simulink model "model"  (R2020b)
settings: Solver=VariableStepAuto  StartTime=0.0  StopTime=20  MaxStep=0.001  RelTol=1e-3
model workspace (MAT data in the model file):
  M1 = Simulink.Parameter
  M1.Value = 100
  M1.DataType = 'auto'
  M1.Dimensions = [1 1]
  b = Simulink.Parameter
  b.Value = 50
  b.DataType = 'auto'
  b.Dimensions = [1 1]
  k1 = Simulink.Parameter
  k1.Value = 50
  k1.DataType = 'auto'
  k1.Dimensions = [1 1]
settings Model: OrderedModelArguments=off  Creator=Lenovo  LastModifiedBy=Lenovo

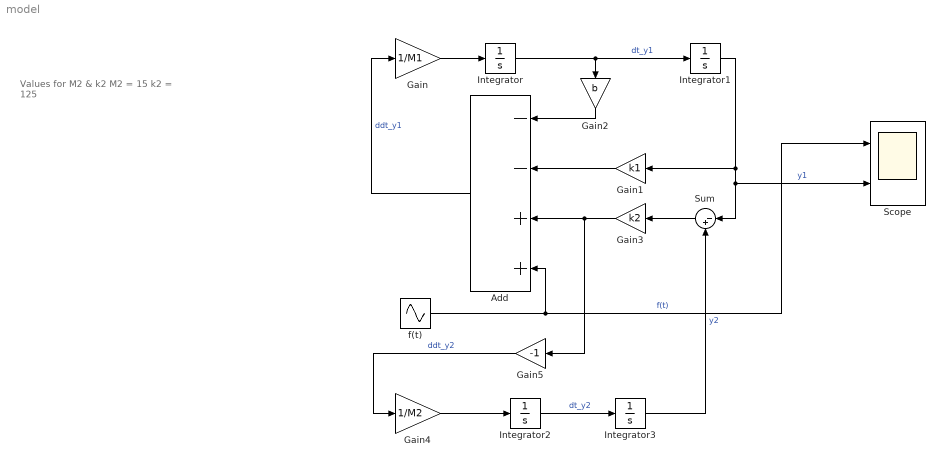
== system model ==
  note: Values for M2 & k2
      | M2 = 15
      | k2 = 125
  Add : Sum  Inputs=--++
  Gain : Gain  Gain=1/M1
  Gain1 : Gain  Gain=k1
  Gain2 : Gain  Gain=b
  Gain3 : Gain  Gain=k2  mask{k2=125}
  Gain4 : Gain  Gain=1/M2  mask{M2=15}
  Gain5 : Gain  Gain=-1
  Integrator{,1..3} (4 alike) : Integrator
  Scope : Scope  NumInputPorts=2
  Sum : Sum  Inputs=|-+
  f(t) : Sin  Amplitude=2  Frequency=10  SampleTime=0
  wires:
  Add/1 -> Gain/1  "ddt_y1"
  Gain/1 -> Integrator/1
  Integrator/1 -> Integrator1/1, Gain2/1  "dt_y1"
  Integrator1/1 -> Scope/2, Sum/1, Gain1/1  "y1"
  Gain2/1 -> Add/1
  Gain1/1 -> Add/2
  Sum/1 -> Gain3/1
  Gain3/1 -> Gain5/1, Add/3
  f(t)/1 -> Add/4, Scope/1  "f(t)"
  Integrator2/1 -> Integrator3/1  "dt_y2"
  Gain4/1 -> Integrator2/1
  Integrator3/1 -> Sum/2  "y2"
  Gain5/1 -> Gain4/1  "ddt_y2"
